simulink model "tf_rl"  (R2022a)
settings: Solver=VariableStepAuto  StartTime=0.0  StopTime=10.0  RelTol=1e-3
libraries: rllib x1
settings Model: Creator=vicky  LastModifiedBy=archi

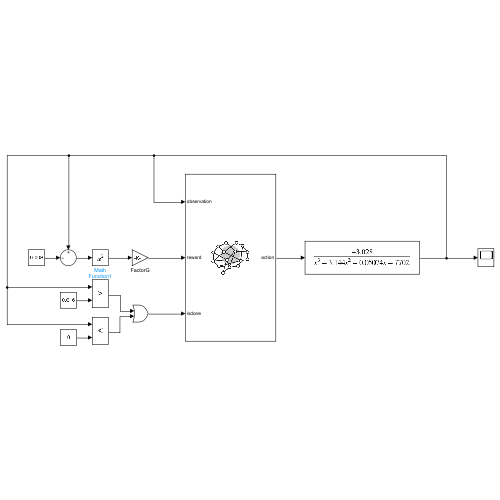
[thumbnail: Simulink's stored preview of the top-level diagram]
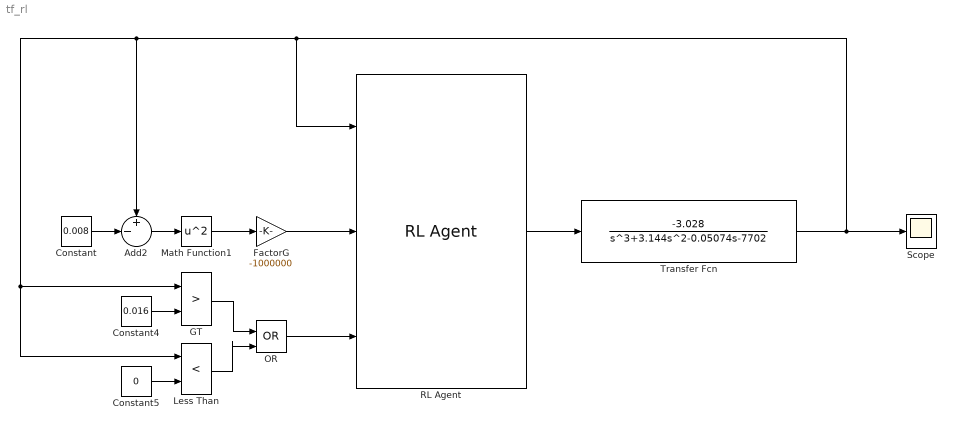
== system tf_rl ==
  Add2 : Sum  Inputs=+-|
  Constant : Constant  Value=0.008
  Constant4 : Constant  Value=0.016
  Constant5 : Constant  Value=0
  FactorG : Gain  Gain=-1000000
  GT : RelationalOperator  Operator=>  OutDataTypeStr=boolean  RndMeth=Simplest  InputSameDT=off
  Less Than : RelationalOperator  Operator=<  OutDataTypeStr=boolean  RndMeth=Simplest  InputSameDT=off
  Math Function1 : Math  Operator=square
  OR : Logic  Operator=OR  IconShape=distinctive  AllPortsSameDT=off  OutDataTypeStr=boolean
  RL Agent : rllib/RL Agent  Agent=rlDDPGAgent  ExternalActionAsInput=off  ProvideLastAction=off  ProvideCumRwd=off  TreatAsDirectFeedthrough=on  UseStrictObservationDataTypes=off
  Scope : Scope
  Transfer Fcn : TransferFcn  Numerator=[-3.028]  Denominator=[1 3.144 -0.05074 -7702]
  wires:
  RL Agent/1 -> Transfer Fcn/1
  Constant/1 -> Add2/2
  Add2/1 -> Math Function1/1
  Math Function1/1 -> FactorG/1
  FactorG/1 -> RL Agent/2
  GT/1 -> OR/1
  Less Than/1 -> OR/2
  Constant4/1 -> GT/2
  Transfer Fcn/1 -> Less Than/1, GT/1, Add2/1, RL Agent/1, Scope/1
  Constant5/1 -> Less Than/2
  OR/1 -> RL Agent/3
